simulink model "powerwindow_org"  (Simulink 10.0)
settings: Solver=FixedStepDiscrete  StartTime=0.0  StopTime=inf  FixedStep=1e-4  RelTol=1e-3  EnableMultiTasking=on
settings Model: Creator=The MathWorks Inc.  LastModifiedBy=bhisma  ExtModeAutoUpdateStatusClock=off
settings DataIOCC: LimitDataPoints=on  SignalLoggingSaveFormat=ModelDataLogs  SignalLoggingName=sigsOut
settings OptimizationCC: BooleanDataType=off  ExpressionDepthLimit=2147483647  InitFltsAndDblsToZero=on
settings DebuggingCC: SaveWithParameterizedLinksMsg=none  SignalResolutionControl=TryResolveAllWithWarning  MultiTaskDSMMsg=warning  MultiTaskCondExecSysMsg=none  FcnCallInpInsideContextMsg=warning  StateNameClashWarn=warning
settings HardwareCC: ProdHWDeviceType=Specified
settings SFSimCC: SimParseCustomCode=off
settings GRTTargetCC: TargetFcnLib=ansi_tfl_tmw.mat  GeneratePreprocessorConditionals=Disable all
settings ConfigComp: CovExternalEMLEnable=off

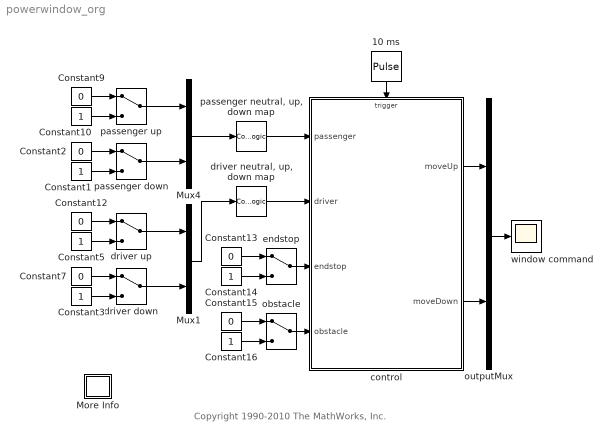
== system powerwindow_org ==
  note: Copyright 1990-2010 The MathWorks, Inc.
  10 ms : DiscretePulseGenerator  PulseType=Time based  Period=1e-2  PulseWidth=50  SampleTime=1e-3
  Constant{1,3,5,10,14,16} (6 alike) : Constant
  Constant{2,7,9,12..13,15} (6 alike) : Constant  Value=0
  More Info : Subsystem
      settings: OpenFcn=showdemo(bdroot(gcb))
      mask Display: disp('?')
  Mux1 : Mux  Inputs=2
  Mux4 : Mux  Inputs=2
  control : Stateflow chart  TreatAsAtomicUnit=on
  "driver neutral, up, down map" : CombinatorialLogic  TruthTable=[1 0 0;0 0 1;0 1 0;1 0 0]
  driver down : ManualSwitch
  driver up : ManualSwitch
  endstop : ManualSwitch
  obstacle : ManualSwitch
  outputMux : Mux  Inputs=2
  "passenger neutral, up, down map" : CombinatorialLogic  TruthTable=[1 0 0;0 0 1;0 1 0;1 0 0]
  passenger down : ManualSwitch
  passenger up : ManualSwitch
  window command : Scope
  wires:
  Constant9/1 -> passenger up/1
  Constant10/1 -> passenger up/2
  Constant2/1 -> passenger down/1
  Constant1/1 -> passenger down/2
  10 ms/1 -> control/Trigger
  passenger down/1 -> Mux4/2
  Constant12/1 -> driver up/1
  Constant5/1 -> driver up/2
  Constant7/1 -> driver down/1
  Constant3/1 -> driver down/2
  driver down/1 -> Mux1/2
  Mux4/1 -> "passenger neutral, up, down map"/1
  Mux1/1 -> "driver neutral, up, down map"/1
  "passenger neutral, up, down map"/1 -> control/1(passenger)
  "driver neutral, up, down map"/1 -> control/2(driver)
  passenger up/1 -> Mux4/1
  driver up/1 -> Mux1/1
  control/1(moveUp) -> outputMux/1
  control/2(moveDown) -> outputMux/2
  outputMux/1 -> window command/1
  Constant13/1 -> endstop/1
  Constant14/1 -> endstop/2
  Constant15/1 -> obstacle/1
  Constant16/1 -> obstacle/2
  endstop/1 -> control/3(endstop)
  obstacle/1 -> control/4(obstacle)

== system powerwindow_org/More Info ==

== stateflow chart control ==
  settings: executeAtInitialization=1
  state safe
    state driverNeutral
      entry:
      moveUp = 0;
      moveDown = 0;
      state passengerneutral
        entry:
        moveUp = 0;
        moveDown = 0;
      state passengerDown
        entry: moveDown = 1;
        exit: moveDown = 0;
        state iniPassengerDown
        state passengerDown
        state autoPassengerDown
        iniPassengerDown -> (junction 41) : after(100,ticks)
        (junction 41) -> autoPassengerDown [order 1] : [passenger[1]]
        (junction 41) -> safe.driverNeutral.passengerDown.passengerDown [order 2]
      state passengerUp
        entry: moveUp = 1;
        exit: moveUp = 0;
        state iniPassengerUp
        state PassengerUp
        state autoPassengerUp
        iniPassengerUp -> (junction 45) : after(100,ticks)
        (junction 45) -> PassengerUp [order 2]
        (junction 45) -> autoPassengerUp [order 1] : [passenger[1]]
      (default) -> passengerneutral
      passengerneutral -> iniPassengerUp [order 1] : [passenger[2]]
      passengerneutral -> iniPassengerDown [order 2] : [passenger[3]]
      safe.driverNeutral.passengerDown.passengerDown -> passengerneutral : [passenger[1]]
      safe.driverNeutral.passengerDown -> passengerneutral [order 1] : [endstop]
      PassengerUp -> passengerneutral : [passenger[1]]
      passengerUp -> passengerneutral [order 2] : [endstop]
      safe.driverNeutral.passengerDown -> PassengerUp [order 2] : [passenger[2]]
      passengerUp -> safe.driverNeutral.passengerDown.passengerDown [order 1] : [passenger[3]]
    state driverDown
      entry: moveDown = 1;
      exit: moveDown = 0;
      state iniDriverDown
      state autoDriverDown
      state DriverDown
      iniDriverDown -> (junction 49) : after(100,ticks)
      (junction 49) -> autoDriverDown [order 1] : [driver[1]]
      (junction 49) -> DriverDown [order 2]
    state driverUp
      entry: moveUp = 1;
      exit: moveUp = 0;
      state iniDriverUp
      state DriverUp
      state autoDriverUp
      iniDriverUp -> (junction 53) : after(100,ticks)
      (junction 53) -> DriverUp [order 2]
      (junction 53) -> autoDriverUp [order 1] : [driver[1]]
    (default) -> driverNeutral
    driverNeutral -> iniDriverDown [order 2] : [driver[3]]
    DriverDown -> driverNeutral : [driver[1]]
    driverDown -> driverNeutral [order 1] : [endstop]
    DriverUp -> driverNeutral : [driver[1]]
    driverUp -> driverNeutral [order 2] : [endstop]
    driverNeutral -> iniDriverUp [order 1] : [driver[2]]
    driverDown -> DriverUp [order 2] : [driver[2]]
    driverUp -> DriverDown [order 1] : [driver[3]]
  state emergencyDown
    entry:
    moveUp = 0;
    moveDown = 1;
  emergencyDown -> passengerneutral : [endstop | after(100,ticks)]
  (default) -> safe
  safe -> emergencyDown : [obstacle]
  data: passenger input boolean size=3; driver input boolean size=3; moveUp output double; moveDown output double; endstop input double; obstacle input double
  events: ticks input RISING_EDGE_EVENT
